simulink model "SpringForce"  (R2026a)
settings: Solver=FixedStepAuto  StopTime=inf
values from neighbouring files (symbols this model uses):
  k = [1.05 0.02 -0.01; 0.03 0.98 0.04; -0.02 0.01 1.02]    [KinematicsTrajectory.m]    (also in Spring.m = 3; SystemModelling.m = 4)
  m = 2    [Spring.m]    (also in SystemModelling.m = 3; pendulumScript.m = 1)
settings Model: Creator=Lenovo LOQ  LastModifiedBy=Lenovo LOQ

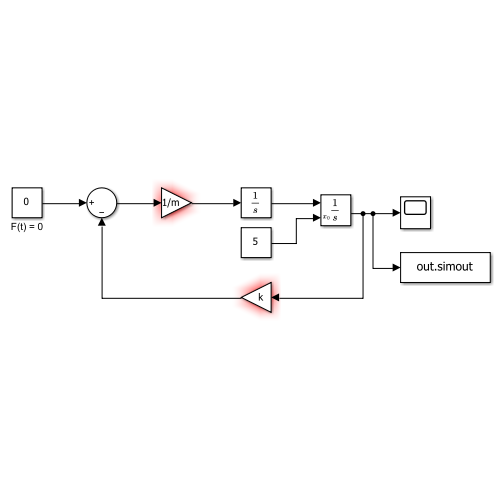
[thumbnail: Simulink's stored preview of the top-level diagram]
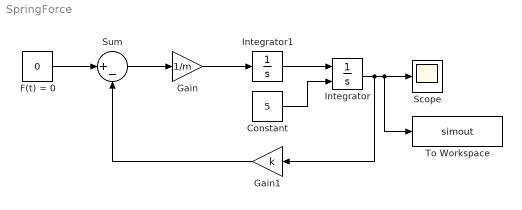
== system SpringForce ==
  Constant : Constant  Value=5
  F(t) = 0 : Constant  Value=0
  Gain : Gain  Gain=1/m
  Gain1 : Gain  Gain=k
  Integrator : Integrator  InitialConditionSource=external
  Integrator1 : Integrator
  Scope : Scope
      settings: ActiveDisplayYMinimum=-1  ActiveDisplayYMaximum=1
  Sum : Sum  Inputs=|+-
  To Workspace : ToWorkspace  VariableName=simout  SaveFormat=Timeseries  SampleTime=-1
  wires:
  Gain/1 -> Integrator1/1
  Sum/1 -> Gain/1
  F(t) = 0/1 -> Sum/1
  Integrator1/1 -> Integrator/1
  Constant/1 -> Integrator/2
  Integrator/1 -> Gain1/1, To Workspace/1, Scope/1
  Gain1/1 -> Sum/2
